simulink model "Tirocinio3Simulink3"  (R2025b)
settings: Solver=VariableStepAuto  StartTime=0.0  StopTime=10.0  RelTol=1e-3
undefined symbols (not defined in the file or in its folder): A_real_system, A_realvals, B_real_system, B_realvals, C_real_system, C_realvals, H_fast_realvals, H_kalman_realvals, H_slow_realvals, M_realvals, R_realvals, V_fast_realvals, V_kalman_realvals, V_slow_realvals
libraries: simulink x1
settings Model: Creator=Davide  LastModifiedBy=Davide

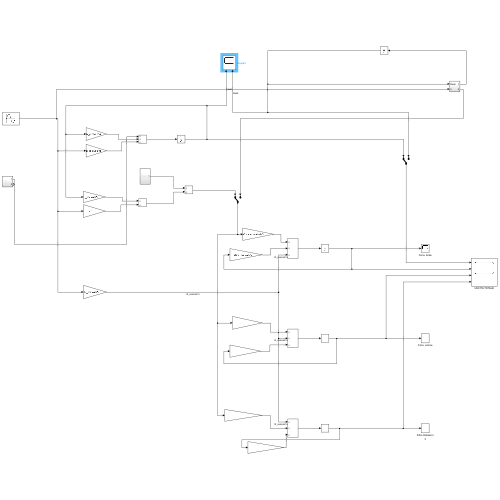
[thumbnail: Simulink's stored preview of the top-level diagram]
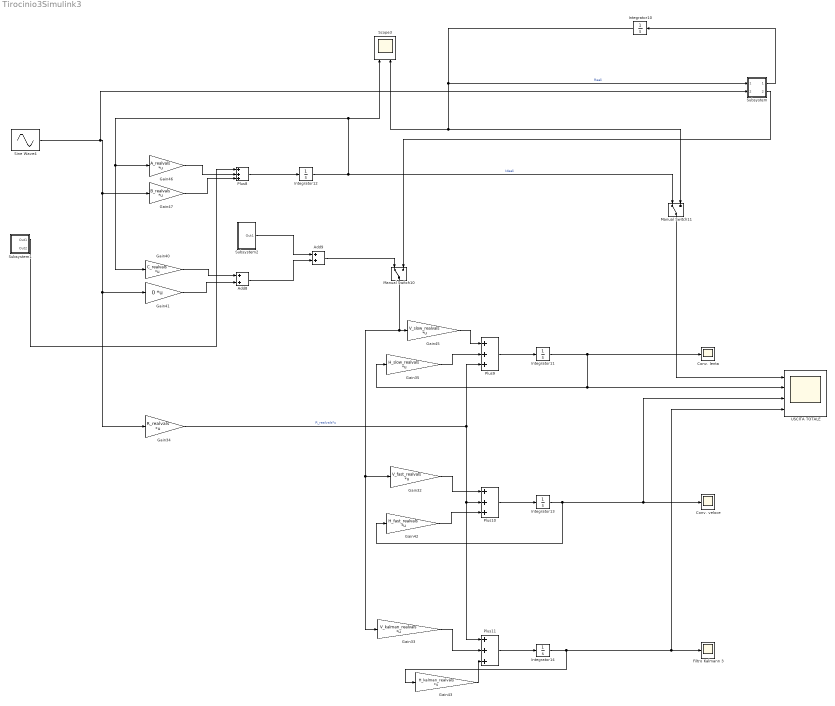
== system Tirocinio3Simulink3 ==
  Add8 : Sum
  Add9 : Sum
  Conv. lenta : Scope
      settings: ActiveDisplayYMinimum=-922.92956  ActiveDisplayYMaximum=1040.41943  DataLoggingVariableName=ScopeData6
  Conv. veloce : Scope
      settings: ActiveDisplayYMinimum=-2.129038696107E+7  ActiveDisplayYMaximum=2.180005183616E+7  DataLoggingVariableName=ScopeData7
  Filtro Kalmann 3 : Scope
      settings: ActiveDisplayYMinimum=-222.82465  ActiveDisplayYMaximum=272.90953  DataLoggingVariableName=ScopeData8
  Gain32 : Gain  Gain=V_fast_realvals  Multiplication=Matrix(K*u)
  Gain33 : Gain  Gain=V_kalman_realvals  Multiplication=Matrix(K*u)
  Gain34 : Gain  Gain=R_realvals  Multiplication=Matrix(K*u)
  Gain35 : Gain  Gain=H_slow_realvals  Multiplication=Matrix(K*u)
  Gain40 : Gain  Gain=C_realvals  Multiplication=Matrix(K*u)
  Gain41 : Gain  Gain=0  Multiplication=Matrix(K*u)
  Gain42 : Gain  Gain=H_fast_realvals  Multiplication=Matrix(K*u)
  Gain43 : Gain  Gain=H_kalman_realvals  Multiplication=Matrix(K*u)
  Gain45 : Gain  Gain=V_slow_realvals  Multiplication=Matrix(K*u)
  Gain46 : Gain  Gain=A_realvals  Multiplication=Matrix(K*u)
  Gain47 : Gain  Gain=B_realvals  Multiplication=Matrix(K*u)
  Integrator10 : Integrator  AbsoluteTolerance=1
  Integrator11 : Integrator  InitialCondition=0.2  AbsoluteTolerance=1
  Integrator12 : Integrator  InitialCondition=0.1  AbsoluteTolerance=1
  Integrator13 : Integrator  InitialCondition=0.2  AbsoluteTolerance=1
  Integrator14 : Integrator  InitialCondition=0.2  AbsoluteTolerance=1
  Manual Switch10 : ManualSwitch
  Manual Switch11 : ManualSwitch
  Plus{8..11} (4 alike) : Sum  Inputs=+++
  Scope3 : Scope  NumInputPorts=2
      settings: ActiveDisplayYMinimum=-1.335137693616405  ActiveDisplayYMaximum=10.69997200714249  DataLoggingVariableName=ScopeData9
  Sine Wave4 : Sin  SampleTime=0
  Subsystem : Subsystem
  Subsystem1 : Subsystem
  Subsystem2 : Subsystem
  "USCITA TOTALE " : Scope  NumInputPorts=4
      settings: ActiveDisplayYMinimum=-1.3290748414179829  ActiveDisplayYMaximum=10.645406337356691  DataLoggingVariableName=ScopeData10
  wires:
  Plus8/1 -> Integrator12/1
  Gain35/1 -> Plus9/2
  Gain40/1 -> Add8/1
  Manual Switch10/1 -> Gain33/1, Gain32/1, Gain45/1
  Plus9/1 -> Integrator11/1
  Plus10/1 -> Integrator13/1
  Gain41/1 -> Add8/2
  Gain32/1 -> Plus10/1
  Gain42/1 -> Plus10/3
  Gain45/1 -> Plus9/1
  Gain43/1 -> Plus11/3
  Sine Wave4/1 -> Subsystem/2(In2), Gain34/1, Gain41/1, Gain47/1
  Integrator12/1 -> Gain40/1, Gain46/1, Scope3/1, Manual Switch11/1  "Ideali"
  Integrator14/1 -> Gain43/1, Filtro Kalmann 3/1, "USCITA TOTALE "/4
  Gain33/1 -> Plus11/2
  Gain34/1 -> Plus9/3, Plus11/1, Plus10/2  "R_realvals*u"
  Integrator10/1 -> Subsystem/1(Reali), Scope3/2, Manual Switch11/2  "Reali"
  Integrator11/1 -> Gain35/1, "USCITA TOTALE "/2, Conv. lenta/1
  Add9/1 -> Manual Switch10/1
  Integrator13/1 -> "USCITA TOTALE "/3, Conv. veloce/1, Gain42/1
  Manual Switch11/1 -> "USCITA TOTALE "/1
  Gain47/1 -> Plus8/3
  Add8/1 -> Add9/2
  Gain46/1 -> Plus8/2
  Plus11/1 -> Integrator14/1
  Subsystem/1(Out1) -> Integrator10/1
  Subsystem/2(Out2) -> Manual Switch10/2
  Subsystem1/1(Out1) -> Plus8/1
  Subsystem2/1(Out1) -> Add9/1

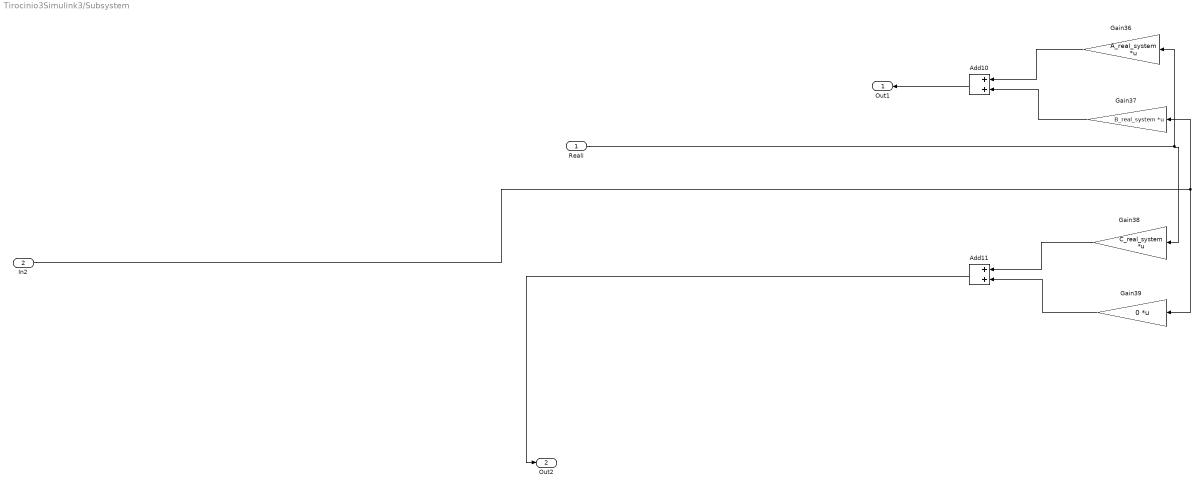
== system Tirocinio3Simulink3/Subsystem ==
  Reali : Inport
  In2 : Inport  Port=2
  Add10 : Sum
  Add11 : Sum
  Gain36 : Gain  Gain=A_real_system  Multiplication=Matrix(K*u)
  Gain37 : Gain  Gain=B_real_system  Multiplication=Matrix(K*u)
  Gain38 : Gain  Gain=C_real_system  Multiplication=Matrix(K*u)
  Gain39 : Gain  Gain=0  Multiplication=Matrix(K*u)
  Out1 : Outport
  Out2 : Outport  Port=2
  wires:
  Add10/1 -> Out1/1
  Gain39/1 -> Add11/2
  Gain37/1 -> Add10/2
  Reali/1 -> Gain38/1, Gain36/1
  Gain36/1 -> Add10/1
  In2/1 -> Gain39/1, Gain37/1
  Gain38/1 -> Add11/1
  Add11/1 -> Out2/1

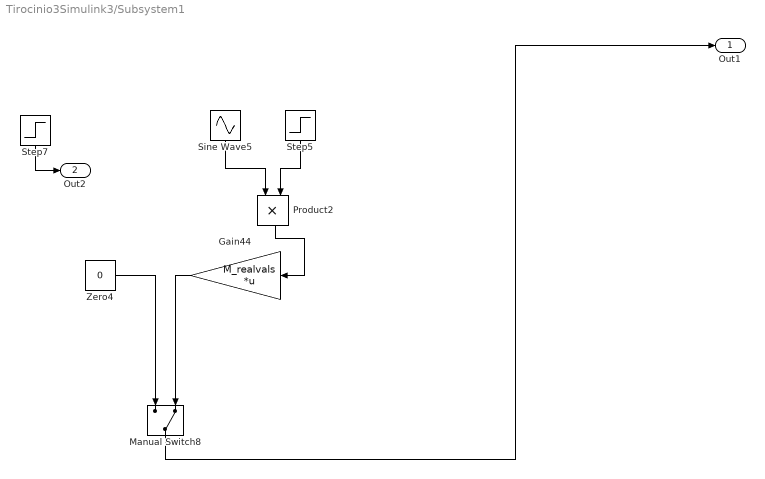
== system Tirocinio3Simulink3/Subsystem1 ==
  Gain44 : Gain  Gain=M_realvals  Multiplication=Matrix(K*u)
  Manual Switch8 : ManualSwitch  CurrentSetting=0
  Product2 : Product
  Sine Wave5 : Sin  SampleTime=0
  Step5 : Step  SampleTime=0
  Step7 : Step  SampleTime=0
  Zero4 : Constant  Value=0  OutDataTypeStr=Inherit: Inherit via back propagation
  Out1 : Outport
  Out2 : Outport  Port=2
  wires:
  Gain44/1 -> Manual Switch8/2
  Step5/1 -> Product2/2
  Sine Wave5/1 -> Product2/1
  Product2/1 -> Gain44/1
  Zero4/1 -> Manual Switch8/1
  Manual Switch8/1 -> Out1/1
  Step7/1 -> Out2/1

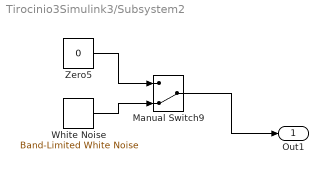
== system Tirocinio3Simulink3/Subsystem2 ==
  Manual Switch9 : ManualSwitch  CurrentSetting=0
  White Noise : simulink/Sources/Band-Limited White Noise  Cov=[10000]  Ts=0.1  seed=[23341]
  Zero5 : Constant  Value=0  OutDataTypeStr=Inherit: Inherit via back propagation
  Out1 : Outport
  wires:
  White Noise/1 -> Manual Switch9/2
  Zero5/1 -> Manual Switch9/1
  Manual Switch9/1 -> Out1/1
